simulink subsystem "battery_charger"  (R2021a)
settings: Solver=VariableStepAuto  StartTime=0.0  StopTime=10.0  RelTol=1e-3
libraries: fl_lib x4, nesl_utility x3, simulink x1
settings Model: Creator=Carlo Edoardo  LastModifiedBy=Carlo Edoardo

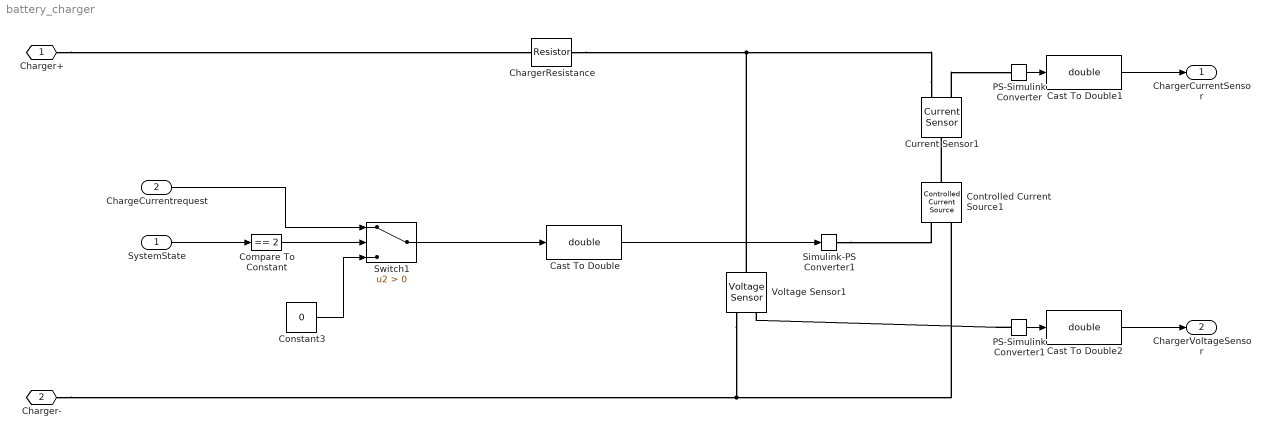
== system battery_charger ==
  SystemState : Inport
  ChargeCurrentrequest : Inport  Port=2
  Cast To Double : DataTypeConversion  OutDataTypeStr=double
  Cast To Double1 : DataTypeConversion  OutDataTypeStr=double
  Cast To Double2 : DataTypeConversion  OutDataTypeStr=double
  ChargerResistance : fl_lib/Electrical/Electrical Elements/Resistor  R=0 Ohm  i_specify=off  i_priority=None  i=0 A  i_nominal_specify=off  i_nominal_unit=A  i_nominal_value=1  v_specify=off  v_priority=None  v=0 V  v_nominal_specify=off  v_nominal_unit=V  v_nominal_value=1
  Compare To Constant : simulink/Logic and Bit Operations/Compare To Constant  relop===  const=2  OutDataTypeStr=boolean
  Constant3 : Constant  Value=0
  Controlled Current Source1 : fl_lib/Electrical/Electrical Sources/Controlled Current Source
  Current Sensor1 : fl_lib/Electrical/Electrical Sensors/Current Sensor
  PS-Simulink Converter : nesl_utility/PS-Simulink Converter  PhysicalDomain=network_engine_domain  SubClassName=ps_output  LeftPortType=input  RightPortType=output  PseudoPeriodic=off  Frequencies=[]  Unit=inherit  AffineConversion=off
      settings: SourceProductBaseCode=PW,SS
  PS-Simulink Converter1 : nesl_utility/PS-Simulink Converter  PhysicalDomain=network_engine_domain  SubClassName=ps_output  LeftPortType=input  RightPortType=output  PseudoPeriodic=off  Frequencies=[]  Unit=inherit  AffineConversion=off
      settings: SourceProductBaseCode=PW,SS
  Simulink-PS Converter1 : nesl_utility/Simulink-PS Converter  PhysicalDomain=network_engine_domain  SubClassName=ps_input  LeftPortType=input  RightPortType=output  PseudoPeriodic=off  Frequencies=[]  NoiseDistribution=none  NoiseParameters=[]  Unit=1  AffineConversion=off  FilteringAndDerivatives=provide  SimscapeFilterOrder=1  InputFilterTimeConstant=0.001  UdotUserProvided=0
      settings: SourceProductBaseCode=PW,SS
  Switch1 : Switch  Criteria=u2 > Threshold
  Voltage Sensor1 : fl_lib/Electrical/Electrical Sensors/Voltage Sensor
  Charger+ : PMIOPort  Side=Left
  Charger- : PMIOPort  Port=2  Side=Left
  ChargerCurrentSensor : Outport
  ChargerVoltageSensor : Outport  Port=2
  wires:
  SystemState/1 -> Compare To Constant/1
  Constant3/1 -> Switch1/3
  Switch1/1 -> Cast To Double/1
  Cast To Double/1 -> Simulink-PS Converter1/1
  ChargeCurrentrequest/1 -> Switch1/1
  Compare To Constant/1 -> Switch1/2
  PS-Simulink Converter/1 -> Cast To Double1/1
  Cast To Double1/1 -> ChargerCurrentSensor/1
  Cast To Double2/1 -> ChargerVoltageSensor/1
  PS-Simulink Converter1/1 -> Cast To Double2/1
  connections:
  Current Sensor1/RConn2 -- Voltage Sensor1/LConn1 -- ChargerResistance/RConn1
  Voltage Sensor1/RConn2 -- Charger-/RConn1 -- Controlled Current Source1/RConn2
  Simulink-PS Converter1/RConn1 -- Controlled Current Source1/RConn1
  Controlled Current Source1/LConn1 -- Current Sensor1/LConn1
  Charger+/RConn1 -- ChargerResistance/LConn1
  Current Sensor1/RConn1 -- PS-Simulink Converter/LConn1
  PS-Simulink Converter1/LConn1 -- Voltage Sensor1/RConn1
